simulink model "interleaver"  (R2020b)
settings: Solver=VariableStepAuto  StartTime=0.0  StopTime=total_time  RelTol=1e-3
values from neighbouring files (symbols this model uses):
  col = 32    [main.m]    (also in parameter.m)
  data_rate = 1000    [parameter.m]
  row = 512    [main.m]    (also in parameter.m)
libraries: commblkintrlv2 x1, commseqgen3 x1
settings Model: Creator=ASUS  LastModifiedBy=ASUS

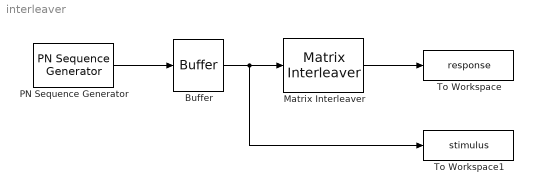
== system interleaver ==
  Buffer : Buffer  N=row*col  OutputFrames=off
  Matrix Interleaver : commblkintrlv2/Matrix Interleaver  StatePerturbationForJacobian=1.0e-05  Nrows=row  Ncols=col
      settings: SourceProductBaseCode=CM
  PN Sequence Generator : commseqgen3/PN Sequence Generator  poly=ploy_PN  ini_sta=seed  outBitMaskSource=Dialog parameter  shift=0  outVarSiz=off  maxOutSizeMode=Dialog parameter  maxOutSize=[10 1]  Ts=1/data_rate  sampPerFrame=1  reset=off  bitPackedOutputs=off  outDataType=boolean  numPackedBits=8  bitPackDataSigned=off  bitPackedOutDType=double
  To Workspace : ToWorkspace  VariableName=response  SampleTime=-1
      settings: Save2DSignal=2-D array (concatenate along first dimension)
  To Workspace1 : ToWorkspace  VariableName=stimulus  SampleTime=-1
      settings: Save2DSignal=2-D array (concatenate along first dimension)
  wires:
  Matrix Interleaver/1 -> To Workspace/1
  PN Sequence Generator/1 -> Buffer/1
  Buffer/1 -> To Workspace1/1, Matrix Interleaver/1
